simulink model "TP2_varying"  (R2020b)
settings: Solver=VariableStepAuto  StartTime=0.0  StopTime=10.0  RelTol=1e-3
values from neighbouring files (symbols this model uses):
  K = lqrd(A,B,Q,R)    [TP2.m]
undefined symbols (not defined in the file or in its folder): A, B, C
libraries: cstblocks x2
settings Model: Creator=João  LastModifiedBy=pedroian

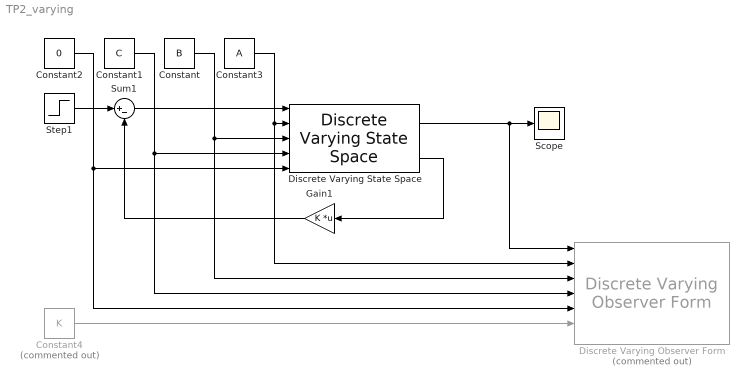
== system TP2_varying ==
  Constant : Constant  Value=B
  Constant1 : Constant  Value=C
  Constant2 : Constant  Value=0
  Constant3 : Constant  Value=A
  Constant4 : Constant  Commented=on  Value=K
  Discrete Varying Observer Form : cstblocks/Linear Parameter Varying/Discrete Varying Observer Form  Commented=on  x0=0  Ts=-1  OutputX=on  OutputDX=on
      settings: SourceProductBaseCode=CT
  Discrete Varying State Space : cstblocks/Linear Parameter Varying/Discrete Varying State Space  x0=0  Ts=0.01  OutputX=on  OutputDX=off
      settings: SourceProductBaseCode=CT
  Gain1 : Gain  Gain=K  Multiplication=Matrix(K*u)
  Scope : Scope
  Step1 : Step  After=10  SampleTime=0
  Sum1 : Sum  Inputs=|+-
  wires:
  Step1/1 -> Sum1/1
  Discrete Varying State Space/2 -> Gain1/1
  Gain1/1 -> Sum1/2
  Sum1/1 -> Discrete Varying State Space/1
  Constant3/1 -> Discrete Varying Observer Form/2, Discrete Varying State Space/2
  Constant2/1 -> Discrete Varying Observer Form/5, Discrete Varying State Space/5
  Constant1/1 -> Discrete Varying Observer Form/4, Discrete Varying State Space/4
  Constant/1 -> Discrete Varying Observer Form/3, Discrete Varying State Space/3
  Discrete Varying State Space/1 -> Scope/1, Discrete Varying Observer Form/1
  Constant4/1 -> Discrete Varying Observer Form/6
